simulink model "MatLab - Simulink - CapstoneWirelessChargerSafety"  (R2025b)
settings: Solver=VariableStepAuto  StartTime=0.0  StopTime=10.0  RelTol=1e-3
undefined symbols (not defined in the file): Ion, Lithium
libraries: spsGroundLib x2, simulink x2, spsBatteryLib x2, spsVariableCapacitorLib x1, spsMutualInductanceLib x1, spsCurrentMeasurementLib x1, spsControlledVoltageSourceLib x1, spsIdealSwitchLib x1, spsUniversalBridgeLib x1, spsVoltageMeasurementLib x1, sps_lib x1
settings Model: Creator=adamn

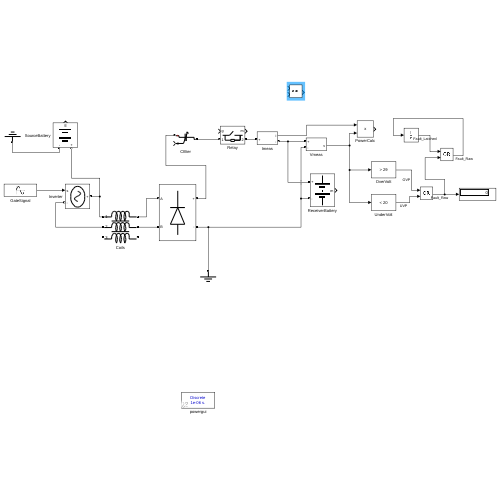
[thumbnail: Simulink's stored preview of the top-level diagram]
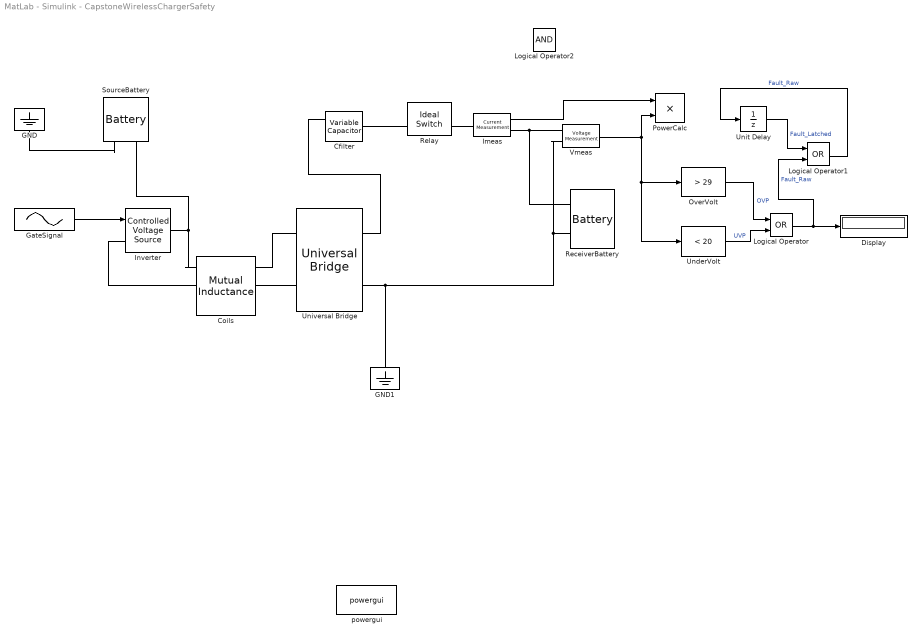
== system MatLab - Simulink - CapstoneWirelessChargerSafety ==
  Cfilter : spsVariableCapacitorLib/Variable Capacitor  methode=Backward Euler  Cabsmin=1e-9  Initialize=off  vC0=0  C0=470e-6  iC0=0
      settings: LibrarySourceBlock=sps_lib/Passives/Variable Capacitor
  Coils : spsMutualInductanceLib/Mutual Inductance  LConnTagsString=a|b|c  RConnTagsString=A|B|C  TypeOfMutual=Two or three windings with equal mutual terms  NumberOfWindings=2  SelfImpedance1=[0.0001 0]  SelfImpedance2=[0.0001 0]  ThreeWindings=on  SelfImpedance3=[ 1.1 1.1e-03]  MutualImpedance=[6e-05 6e-05]  InductanceMatrix="[1.0 0.9  0.9 ;  0.9 1.0  0.9;  0.9 0.9 1.0 ] * 1e-3"  ResistanceMatrix="[1.0 0.9  0.9 ;  0.9 1.0  0.9;  0.9 0.9 1.0 ]"  Measurements=None
      settings: LibrarySourceBlock=sps_lib/Passives/Mutual Inductance
  Display : Display
  GND : spsGroundLib/Ground  LConnTagsString=a
  GND1 : spsGroundLib/Ground  LConnTagsString=a
  GateSignal : Sin  Frequency=20000  SampleTime=0
  Imeas : spsCurrentMeasurementLib/Current Measurement  PhasorSimulation=off  OutputType=Complex  PSBequivalent=0
  Inverter : spsControlledVoltageSourceLib/Controlled Voltage Source  Initialize=on  Source_Type=AC  Amplitude=0  Phase=0  Frequency=0  Measurements=None
  Logical Operator : Logic  Operator=OR  AllPortsSameDT=off  OutDataTypeStr=boolean
  Logical Operator1 : Logic  Operator=OR  AllPortsSameDT=off  OutDataTypeStr=boolean
  Logical Operator2 : Logic  AllPortsSameDT=off  OutDataTypeStr=boolean
  OverVolt : simulink/Logic and Bit Operations/Compare To Constant  relop=>  const=29  OutDataTypeStr=boolean
  PowerCalc : Product  Inputs=**
  ReceiverBattery : spsBatteryLib/Battery  BatType=Lithium-Ion  NomV=25.6  NomQ=100  SOC=0.9  Batt_Tr=30  PresetModel=on  MaxQ=100  MinV=19.2  FullV=29.7981  Dis_rate=43.4783  R=0.00256  Normal_OP=90.4348  expZone="[27.6579      4.91304]"
  Relay : spsIdealSwitchLib/Ideal Switch  Ron=0.001  Lon=0  IC=0  Rs=1e5  Cs=inf  Measurements=on
  SourceBattery : spsBatteryLib/Battery  BatType=Lithium-Ion  NomV=24  NomQ=100  SOC=0.9  Batt_Tr=30  PresetModel=on  MaxQ=100  MinV=18  FullV=27.9357  Dis_rate=43.4783  R=0.0024  Normal_OP=90.4348  expZone="[25.9293      4.91304]"
  UnderVolt : simulink/Logic and Bit Operations/Compare To Constant  relop=<  const=20  OutDataTypeStr=boolean
  Unit Delay : UnitDelay  SampleTime=-1  HasFrameUpgradeWarning=on
  Universal Bridge : spsUniversalBridgeLib/Universal Bridge  Arms=2  SnubberResistance=1e5  SnubberCapacitance=inf  Device=Diodes  Ron=1e-3  Lon=0  ForwardVoltages="[  0  0  ]"  ForwardVoltage=0  GTOparameters=[ 10e-6 , 20e-6 ]  IGBTparameters=[ 1e-6 , 2e-6 ]  Measurements=None  Measurements_2=None  converterType=Rectifier
  Vmeas : spsVoltageMeasurementLib/Voltage Measurement  PhasorSimulation=off  OutputType=Complex  PSBequivalent=0
  powergui : sps_lib/powergui  Priority=1  SimulationMode=Discrete  SampleTime=1e-6  frequency=60  Iterations=50  frequencyindice=0  Pbase=100e6  ErrMax=1e-4  UnitsV=kV  UnitsW=MW  buscounter=0  FunctionMessages=off  echomessages=off  EnableUseOfTLC=off  CurrentSourceSwitches=off  DisableSnubberDevices=off  DisableRonSwitches=off  DisableVfSwitches=off  DisplayEquations=off  AutomaticDiscreteSolvers=off  SolverType=Tustin/Backward Euler (TBE)  Interpol=off  ExternalGateDelay=off  methode=off  Ts=100  x0status=blocks  SPID=on  SwTol=0  HookPort=off  NonlinearTolerance=1e-4  nMaxIteration=100  ContinueOnMaxIteration=off  RestoreLinks=warning  ResistiveCurrentMeasurement=off  Frange=[0:2:500]  Ylog=off  Xlog=on  ShowGrid=off  save=off  variable=ZData  structure=0  ZoomFFT=off  StartTime=0.0  cycles=1  DisplayStyle=1  fundamental=60  FreqAxis=off  MaxFrequency=1000  frequencyindicesteady=1  RmsSteady=1  display=off
  wires:
  GateSignal/1 -> Inverter/1
  Vmeas/1 -> UnderVolt/1, OverVolt/1, PowerCalc/2
  Imeas/1 -> PowerCalc/1
  OverVolt/1 -> Logical Operator/1  "OVP"
  UnderVolt/1 -> Logical Operator/2  "UVP"
  Logical Operator/1 -> Logical Operator1/2, Display/1  "Fault_Raw"
  Unit Delay/1 -> Logical Operator1/1  "Fault_Latched"
  Logical Operator1/1 -> Unit Delay/1  "Fault_Raw"
  connections:
  SourceBattery/LConn1 -- Coils/LConn1 -- Inverter/RConn1
  SourceBattery/LConn2 -- GND/LConn1
  Inverter/LConn1 -- Coils/LConn2
  Coils/RConn1 -- Universal Bridge/LConn1
  Coils/RConn2 -- Universal Bridge/LConn2
  Universal Bridge/RConn1 -- Cfilter/LConn1
  ReceiverBattery/LConn1 -- Vmeas/LConn1 -- Imeas/RConn1
  ReceiverBattery/LConn2 -- Universal Bridge/RConn2 -- GND1/LConn1 -- Vmeas/LConn2
  Cfilter/RConn1 -- Relay/LConn1
  Relay/RConn1 -- Imeas/LConn1
